simulink model "guidepathtracking"  (Simulink 6.2)
settings: Solver=ode3  StartTime=0.0  StopTime=10  FixedStep=.05  RelTol=1e-4
libraries: simulink x1
settings Model: Creator=diduch  LastModifiedBy=diduch
settings DebuggingCC: SignalResolutionControl=UseLocalSettings  SolverPrmCheckMsg=warning  MultiTaskDSMMsg=error

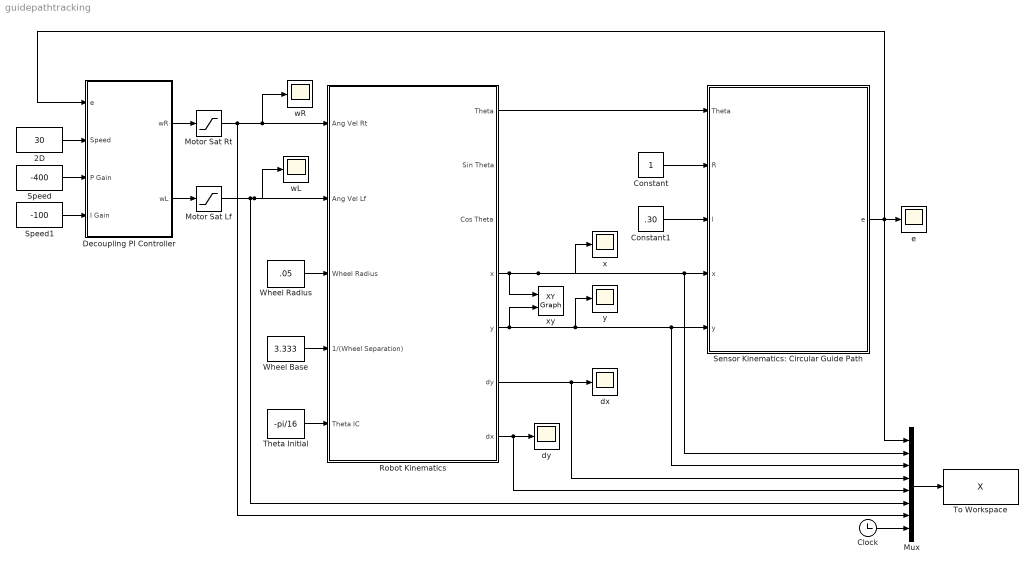
== system guidepathtracking ==
  2D : Constant  Value=30
  Clock : Clock
      settings: Decimation=10
  Constant : Constant
  Constant1 : Constant  Value=.30
  Decoupling PI Controller : Subsystem
  Motor Sat Lf : Saturate  UpperLimit=100*pi  LowerLimit=-100*pi
  Motor Sat Rt : Saturate  UpperLimit=100*pi  LowerLimit=-100*pi
  Mux : Mux  Inputs=8
  Robot Kinematics : Subsystem
  Sensor Kinematics: Circular Guide Path : Stateflow chart
  Speed : Constant  Value=-400
  Speed1 : Constant  Value=-100
  Theta Initial : Constant  Value=-pi/16  VectorParams1D=off  OutDataTypeMode=double
  To Workspace : ToWorkspace  VariableName=X  SampleTime=-1  SaveFormat=Array
  Wheel Base : Constant  Value=3.333
  Wheel Radius : Constant  Value=.05
  dx : Scope
      settings: TimeRange=2.8  YMin=-39.94478527607363  YMax=4.055214723926369  SaveName=ScopeData11
  dy : Scope
      settings: TimeRange=2.8  YMin=-39.94478527607363  YMax=4.055214723926369  SaveName=ScopeData12
  e : Scope
      settings: TimeRange=2.8  YMin=-39.94478527607363  YMax=4.055214723926369
  wL : Scope
      settings: TimeRange=2  YMin=313  YMax=316  SaveName=ScopeData2
  wR : Scope
      settings: YMin=-50  YMax=350
  x : Scope
      settings: TimeRange=2.8  YMin=-39.94478527607363  YMax=4.055214723926369  SaveName=ScopeData4
  xy : simulink/Sinks/XY Graph  xmin=-2  xmax=2  ymin=-2  ymax=2  st=-1
  y : Scope
      settings: TimeRange=2.8  YMin=-39.94478527607363  YMax=4.055214723926369  SaveName=ScopeData5
  wires:
  Wheel Radius/1 -> Robot Kinematics/3(Wheel Radius)
  Wheel Base/1 -> Robot Kinematics/4(1/(Wheel Separation))
  Theta Initial/1 -> Robot Kinematics/5(Theta IC)
  Robot Kinematics/5(y) -> xy/2, y/1, Sensor Kinematics: Circular Guide Path/5(y), Mux/3
  Robot Kinematics/4(x) -> xy/1, x/1, Sensor Kinematics: Circular Guide Path/4(x), Mux/2
  Robot Kinematics/1(Theta) -> Sensor Kinematics: Circular Guide Path/1(Theta)
  Motor Sat Lf/1 -> Robot Kinematics/2(Ang Vel Lf), wL/1, Mux/6
  Constant/1 -> Sensor Kinematics: Circular Guide Path/2(R)
  Constant1/1 -> Sensor Kinematics: Circular Guide Path/3(l)
  Sensor Kinematics: Circular Guide Path/1(e) -> Decoupling PI Controller/1(e), e/1, Mux/1
  Robot Kinematics/6(dy) -> dx/1, Mux/4
  Robot Kinematics/7(dx) -> dy/1, Mux/5
  2D/1 -> Decoupling PI Controller/2(Speed)
  Speed/1 -> Decoupling PI Controller/3(P Gain)
  Decoupling PI Controller/1(wR) -> Motor Sat Rt/1
  Decoupling PI Controller/2(wL) -> Motor Sat Lf/1
  Speed1/1 -> Decoupling PI Controller/4(I Gain)
  Motor Sat Rt/1 -> Robot Kinematics/1(Ang Vel Rt), wR/1, Mux/7
  Mux/1 -> To Workspace/1
  Clock/1 -> Mux/8

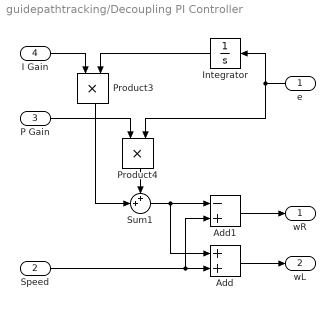
== system guidepathtracking/Decoupling PI Controller ==
  e : Inport  Orientation=left  Port=1  LatchInput=off
  Speed : Inport  Port=2  LatchInput=off
  P Gain : Inport  Port=3  LatchInput=off
  I Gain : Inport  Port=4  LatchInput=off
  Add : Sum  OutScaling=2^-10
  Add1 : Sum  Inputs=-+  OutScaling=2^-10
  Integrator : Integrator  Orientation=left
  Product3 : Product  Orientation=down  RndMeth=Zero
  Product4 : Product  Orientation=down  RndMeth=Zero
  Sum1 : Sum  Inputs=++|
  wR : Outport
  wL : Outport  Port=2
  wires:
  Add/1 -> wL/1
  Add1/1 -> wR/1
  e/1 -> Integrator/1, Product4/2
  I Gain/1 -> Product3/1
  Integrator/1 -> Product3/2
  P Gain/1 -> Product4/1
  Product4/1 -> Sum1/1
  Product3/1 -> Sum1/2
  Sum1/1 -> Add1/1, Add/1
  Speed/1 -> Add/2, Add1/2

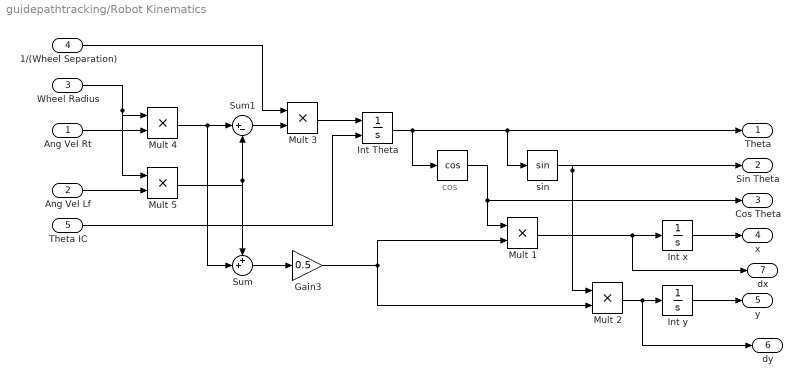
== system guidepathtracking/Robot Kinematics ==
  note: cos
  Ang Vel Rt : Inport  Port=1  LatchInput=off
  Ang Vel Lf : Inport  Port=2  LatchInput=off
  Wheel Radius : Inport  Port=3  LatchInput=off
  1/(Wheel Separation) : Inport  Port=4  LatchInput=off
  Theta IC : Inport  Port=5  LatchInput=off
  " " : Trigonometry  Operator=cos
  Gain3 : Gain  Gain=0.5
  Int Theta : Integrator  InitialConditionSource=external  InitialCondition=1  ZeroCross=off
  Int x : Integrator
  Int y : Integrator  InitialCondition=-1.1
  Mult {1..5} (5 alike) : Product  RndMeth=Zero
  Sum : Sum  Inputs=++|
  Sum1 : Sum  Inputs=|+-
  sin : Trigonometry
  Theta : Outport
  Sin Theta : Outport  Port=2
  Cos Theta : Outport  Port=3
  x : Outport  Port=4
  y : Outport  Port=5
  dy : Outport  Port=6
  dx : Outport  Port=7
  wires:
  Mult 4/1 -> Sum1/1, Sum/2
  Mult 5/1 -> Sum1/2, Sum/1
  Sum1/1 -> Mult 3/2
  Sum/1 -> Gain3/1
  Int Theta/1 -> " "/1, sin/1, Theta/1
  Gain3/1 -> Mult 1/2, Mult 2/2
  " "/1 -> Mult 1/1, Cos Theta/1
  Mult 1/1 -> Int x/1, dx/1
  Mult 2/1 -> Int y/1, dy/1
  sin/1 -> Mult 2/1, Sin Theta/1
  Int x/1 -> x/1
  Int y/1 -> y/1
  Mult 3/1 -> Int Theta/1
  Ang Vel Lf/1 -> Mult 5/2
  Ang Vel Rt/1 -> Mult 4/2
  Wheel Radius/1 -> Mult 4/1, Mult 5/1
  1/(Wheel Separation)/1 -> Mult 3/1
  Theta IC/1 -> Int Theta/2

== matlab function Sensor Kinematics: Circular Guide Path ==
  data: Theta input inherited; R input inherited; l input inherited; x input inherited; y input inherited; e output inherited
function e = CircularGuidePath(Theta,R,l,x,y)
% C.P. Diduch, February 16, 2013
% l: distance from vehicle centre to centre of linear optical array
% R: radius of guidpath - guidepath is a circle centred at (0, 0)
% [x, y, Theta]: robot pose
% e: distance from the centre of the sensor to the guidepath and
% perpendicular to the vehicle orientation, Theta.

b=2*(y*cos(Theta)-x*sin(Theta));
c=x^2+y^2-R^2+l^2+2*l*(x*cos(Theta)+y*sin(Theta));
z=b^2-4*c;
if(z>0) % If there are 2 solutions:
    e1=0.5*(-b+sqrt(z));
    e2=0.5*(-b-sqrt(z));
else % If there are no solutions return an 'arbitrary' value (with z=0):
    e1=-0.5*b;
    e2=e1;
end
%e=[e1;e2];
if(abs(e1)<abs(e2))e=e1;
else e=e2;
end
